simulink model "practica1_ej1_simulink"  (R2022b)
settings: Solver=VariableStepAuto  StartTime=0.0  StopTime=120.0  RelTol=1e-3
settings Model: Creator=Usuario_UMA  LastModifiedBy=Usuario_UMA

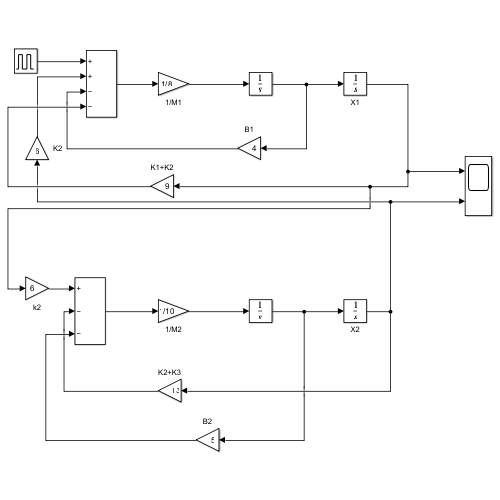
[thumbnail: Simulink's stored preview of the top-level diagram]
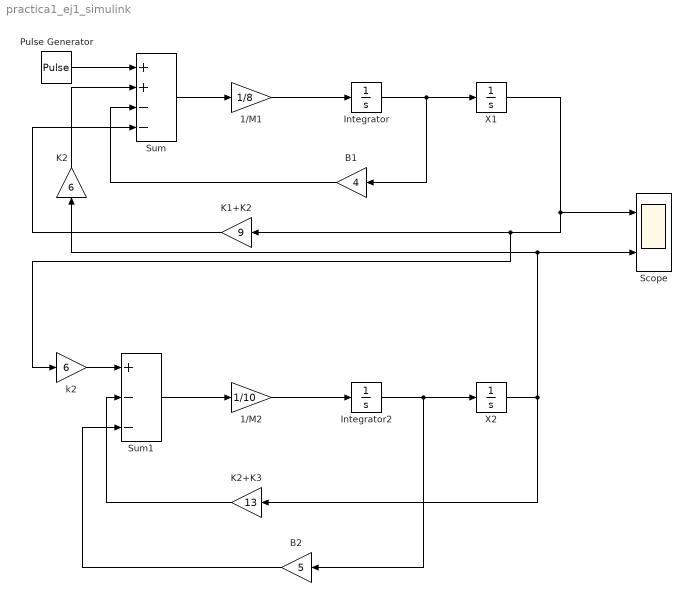
== system practica1_ej1_simulink ==
  1/M1 : Gain  Gain=1/8
  1/M2 : Gain  Gain=1/10
  B1 : Gain  Gain=4
  B2 : Gain  Gain=5
  Integrator : Integrator
  Integrator2 : Integrator
  K1+K2 : Gain  Gain=9
  K2 : Gain  Gain=6
  K2+K3 : Gain  Gain=13
  Pulse Generator : DiscretePulseGenerator  PulseType=Time based  Period=50  PulseWidth=20
  Scope : Scope  NumInputPorts=2
  Sum : Sum  Inputs=++--
  Sum1 : Sum  Inputs=+--
  X1 : Integrator
  X2 : Integrator
  k2 : Gain  Gain=6
  wires:
  Pulse Generator/1 -> Sum/1
  K2/1 -> Sum/2
  Sum/1 -> 1/M1/1
  1/M1/1 -> Integrator/1
  Integrator/1 -> B1/1, X1/1
  X1/1 -> k2/1, K1+K2/1, Scope/1
  B1/1 -> Sum/3
  K1+K2/1 -> Sum/4
  1/M2/1 -> Integrator2/1
  Integrator2/1 -> B2/1, X2/1
  X2/1 -> K2+K3/1, Scope/2, K2/1
  Sum1/1 -> 1/M2/1
  k2/1 -> Sum1/1
  K2+K3/1 -> Sum1/2
  B2/1 -> Sum1/3
